simulink model "attitude3d"  (R2019b)
settings: Solver=ode4  StartTime=0.0  StopTime=6530  FixedStep=10  RelTol=1e-3
values from neighbouring files (symbols this model uses):
  antenna_vb = [1, 0, 0]    [attitude3d_init.m]
  init_xBI = [1, 0, 0]    [attitude3d_init.m]
  init_yBI = [0, 1, 0]    [attitude3d_init.m]
  init_zBI = [0, 0, 1]    [attitude3d_init.m]
  P = 2 * pi / mean_motion    [attitude3d_init.m]
  solar_array_vb = [1, 0, 0]    [attitude3d_init.m]
  star_sensor_1_vb = [1/sqrt(2), +1/sqrt(2), 0]    [attitude3d_init.m]
  star_sensor_2_vb = [1/sqrt(2), -1/sqrt(2), 0]    [attitude3d_init.m]
  target_mean_radius = mean_mars_radius    (= 3389500)    [attitude3d_init.m]
  thrust_no_shadow_weight = 1.0    (= 1)    [attitude3d_init.m]
  thrust_shadow_weight = 1.0    (= 1)    [attitude3d_init.m]
  thruster_vb = [-1, 0, 0]    [attitude3d_init.m]
  window_n = int16(window_t/10.0)    [attitude3d_init.m]
  x = [0,        max_omega*0.1,  0, 0               ;      0.5 * P,  max_omega*0.1,  0, 0               ;      1.0 * P,  max_omega*0.1,  0, 0               ]    [attitude3d_init.m]
libraries: vrlib x14, simulink x6, dspstat3 x4, commfilt2 x2
(part 1 of 2)
settings Model: Creator=ggarrett  LastModifiedBy=ggarrett
settings HardwareCC: TargetBitPerLong=64  TargetBitPerPointer=64  TargetBitPerSizeT=64  TargetBitPerPtrDiffT=64  TargetLongLongMode=on  TargetIntDivRoundTo=Zero  TargetEndianess=LittleEndian  TargetWordSize=64  TargetHWDeviceType=MATLAB Host  ProdEqTarget=off
settings RTWCC: Description=Rapid Simulation Target  SystemTargetFile=rsim.tlc  TemplateMakefile=rsim_default_tmf
settings RSimTargetCC: TargetLangStandard=C99 (ISO)  GeneratePreprocessorConditionals=Use local settings  PreserveStateflowLocalDataDimensions=off

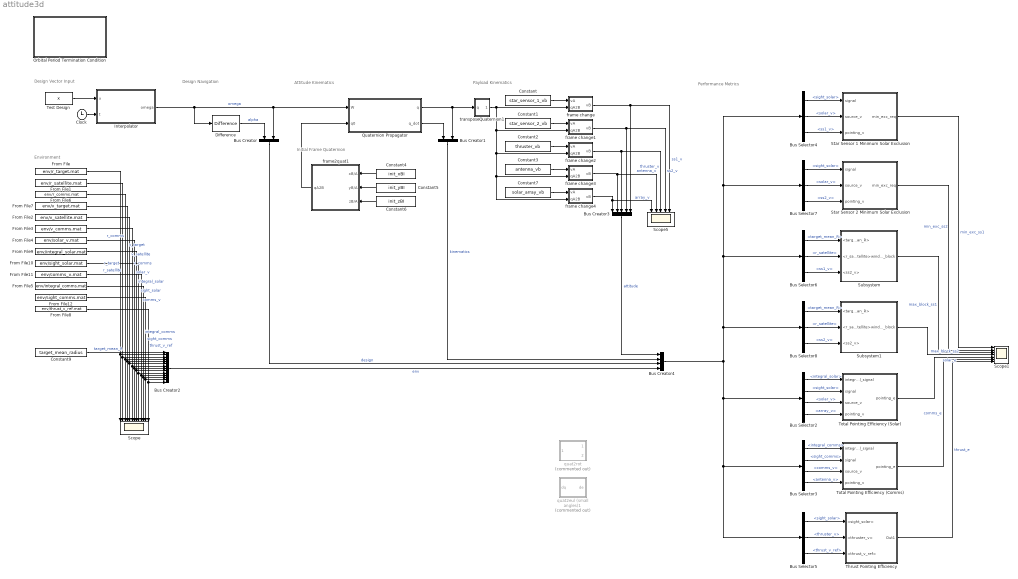
== system attitude3d ==
  note: Performance Metrics
  note: Attitude Kinematics
  note: Design Vector Input
  note: Design Navigation
  note: Payload Kinematics
  note: Environment
  note: Initial Frame Quaternion
  Bus Creator : BusCreator  Inputs=2
  Bus Creator1 : BusCreator  Inputs=2
  Bus Creator2 : BusCreator  Inputs=14
  Bus Creator3 : BusCreator  Inputs=5
  Bus Creator4 : BusCreator  Inputs=4
  Bus Selector2 : BusSelector  OutputSignals=env.integral_solar,env.sight_solar,env.solar_v,attitude.array_v
  Bus Selector3 : BusSelector  OutputSignals=env.integral_comms,env.sight_comms,env.comms_v,attitude.antenna_v
  Bus Selector4 : BusSelector  OutputSignals=env.sight_solar,env.solar_v,attitude.ss1_v
  Bus Selector5 : BusSelector  OutputSignals=env.sight_solar,attitude.thruster_v,env.thrust_v_ref
  Bus Selector6 : BusSelector  OutputSignals=env.target_mean_R,env.r_satellite,attitude.ss1_v
  Bus Selector7 : BusSelector  OutputSignals=env.sight_solar,env.solar_v,attitude.ss2_v
  Bus Selector8 : BusSelector  OutputSignals=env.target_mean_R,env.r_satellite,attitude.ss2_v
  Clock : Clock
  Constant : Constant  Value=star_sensor_1_vb
  Constant1 : Constant  Value=star_sensor_2_vb
  Constant2 : Constant  Value=thruster_vb
  Constant3 : Constant  Value=antenna_vb
  Constant4 : Constant  Value=init_xBI
  Constant5 : Constant  Value=init_yBI
  Constant6 : Constant  Value=init_zBI
  Constant7 : Constant  Value=solar_array_vb
  Constant9 : Constant  Value=target_mean_radius
  Difference : simulink/Discrete/Difference  ICPrevInput=0.0  OutMin=[]  OutMax=[]  OutDataType=fixdt(1, 16)  OutScaling=2^-10  DoSatur=off
  From File : FromFile  FileName=env/r_target.mat  SampleTime=0
  From File1 : FromFile  FileName=env/r_satellite.mat  SampleTime=0
  From File10 : FromFile  FileName=env/sight_solar.mat  SampleTime=0
  From File11 : FromFile  FileName=env/comms_v.mat  SampleTime=0
  From File12 : FromFile  FileName=env/sight_comms.mat  SampleTime=0
  From File2 : FromFile  FileName=env/v_satellite.mat  SampleTime=0
  From File3 : FromFile  FileName=env/v_comms.mat  SampleTime=0
  From File4 : FromFile  FileName=env/solar_v.mat  SampleTime=0
  From File5 : FromFile  FileName=env/integral_comms.mat  SampleTime=0
  From File6 : FromFile  FileName=env/r_comms.mat  SampleTime=0
  From File7 : FromFile  FileName=env/v_target.mat  SampleTime=0
  From File8 : FromFile  FileName=env/thrust_v_ref.mat  SampleTime=0
  From File9 : FromFile  FileName=env/integral_solar.mat  SampleTime=0
  "Interpolator " : MATLAB Function  TreatAsAtomicUnit=on
  Orbital Period Termination Condition : Subsystem
  Quaternion Propagator : Subsystem
  Scope : Scope  NumInputPorts=13
  Scope1 : Scope  NumInputPorts=7
  Scope5 : Scope  NumInputPorts=5
  Star Sensor 1 Minimum Solar Exclusion : Subsystem
  Star Sensor 2 Minimum Solar Exclusion : Subsystem
  Subsystem : Subsystem
  Subsystem1 : Subsystem
  Test Design : Constant  Value=x
  Thrust Pointing Efficiency : Subsystem
  Total Pointing Efficiency (Comms) : Subsystem
  Total Pointing Efficiency (Solar) : Subsystem
  frame change : Subsystem  mask(Frame change){inLabel=b, outLabel=i}
      mask prompts: inLabel "Label for initial frame"; outLabel "Label for target frame"
      mask help: Express input vector in frame B, using the quaternion describing the rotation from frame A to frame B.
      mask Display:
      | port_label('input',1,['v',inLabel]);
      | port_label('output',1,['v',outLabel]);
      | port_label('input',2,['q',inLabel,'2',outLabel]);
  frame change1 : Subsystem  mask(Frame change){inLabel=b, outLabel=i}
      mask prompts: inLabel "Label for initial frame"; outLabel "Label for target frame"
      mask help: Express input vector in frame B, using the quaternion describing the rotation from frame A to frame B.
      mask Display:
      | port_label('input',1,['v',inLabel]);
      | port_label('output',1,['v',outLabel]);
      | port_label('input',2,['q',inLabel,'2',outLabel]);
  frame change2 : Subsystem  mask(Frame change){inLabel=b, outLabel=i}
      mask prompts: inLabel "Label for initial frame"; outLabel "Label for target frame"
      mask help: Express input vector in frame B, using the quaternion describing the rotation from frame A to frame B.
      mask Display:
      | port_label('input',1,['v',inLabel]);
      | port_label('output',1,['v',outLabel]);
      | port_label('input',2,['q',inLabel,'2',outLabel]);
  frame change3 : Subsystem  mask(Frame change){inLabel=b, outLabel=i}
      mask prompts: inLabel "Label for initial frame"; outLabel "Label for target frame"
      mask help: Express input vector in frame B, using the quaternion describing the rotation from frame A to frame B.
      mask Display:
      | port_label('input',1,['v',inLabel]);
      | port_label('output',1,['v',outLabel]);
      | port_label('input',2,['q',inLabel,'2',outLabel]);
  frame change4 : Subsystem  mask(Frame change){inLabel=b, outLabel=i}
      mask prompts: inLabel "Label for initial frame"; outLabel "Label for target frame"
      mask help: Express input vector in frame B, using the quaternion describing the rotation from frame A to frame B.
      mask Display:
      | port_label('input',1,['v',inLabel]);
      | port_label('output',1,['v',outLabel]);
      | port_label('input',2,['q',inLabel,'2',outLabel]);
  frame2quat1 : Subsystem  mask(Compute quaternion from 3 orthogonal unit vectors){Alabel=I, Blabel=B}
      mask prompts: Alabel "Label for origin frame"; Blabel "Label for target frame"
      mask help: Determines the attitude quaternion representing the rotation which transforms the origin frame into the target frame, from the unit vectors of target frame expressed in origin frame.
      mask Display:
      | port_label('input',1,['x',Blabel,'/',Alabel]);
      | port_label('input',2,['y',Blabel,'/',Alabel]);
      | port_label('input',3,['z',Blabel,'/',Alabel]);
      | port_label('output',1,['q',Alabel,'2',Blabel]);
  quat2eul (small angles)1 : Subsystem  Commented=on  mask(Small quat error to small angles error){}
      mask help:
      | [dphi,dtheta,dpsi] = u*dTheta
      | where
      | dq = [cos(dTheta/2); u*sin(dTheta/2)]
  quat2rot : Subsystem  Commented=on  mask(Find axis and angle from quaternion){Alabel=I, Blabel=B}
      mask prompts: Alabel "Label for origin frame"; Blabel "Label for target frame"
      mask help: Extracts the axis (unit vector) and angle (rad) of the rotation from origin frame to target frame, from the quaternion representing that rotation
      mask Display:
      | port_label('input',1,['q',Alabel,'2',Blabel]);
      | port_label('output',1,['th_',Alabel,'2',Blabel]);
      | port_label('output',2,['u_',Alabel]);
  transposeQuaternion1 : Subsystem  mask(transposeQuaternion){}
      mask help:
      | Compute the transpose (inverse or conjugate) of the input quaternion
      |
      | Inputs:
      |   q     Quaternion
      |
      | Outputs:
      |   qt     Transpose of the input quaternion
      mask Help: eval('starDoc simulink/transposeQuaternion');
      mask Display: disp('q''');
  wires:
  Test Design/1 -> "Interpolator "/1(x)
  Clock/1 -> "Interpolator "/2(t)
  From File/1 -> Scope/1, Bus Creator2/2  "r_target"
  From File1/1 -> Scope/2, Bus Creator2/3  "r_satellite"
  From File6/1 -> Scope/3, Bus Creator2/4  "r_comms"
  From File7/1 -> Scope/4, Bus Creator2/5  "v_target"
  From File2/1 -> Scope/5, Bus Creator2/6  "v_satellite"
  From File3/1 -> Scope/6, Bus Creator2/7  "v_comms"
  From File4/1 -> Scope/7, Bus Creator2/8  "solar_v"
  "Interpolator "/1(omega) -> Difference/1, Quaternion Propagator/1(W), Bus Creator/2  "omega"
  Difference/1 -> Bus Creator/1  "alpha"
  Quaternion Propagator/2(q_dot) -> Bus Creator1/1
  Constant/1 -> frame change/1(vA)
  Constant1/1 -> frame change1/1(vA)
  Constant2/1 -> frame change2/1(vA)
  Constant3/1 -> frame change3/1(vA)
  Bus Creator/1 -> Bus Creator4/3  "design"
  Bus Creator1/1 -> Bus Creator4/2  "kinematics"
  Bus Creator2/1 -> Bus Creator4/4  "env"
  Constant5/1 -> frame2quat1/2(yB/A)
  Quaternion Propagator/1(q) -> transposeQuaternion1/1(q), Bus Creator1/2
  Constant6/1 -> frame2quat1/3(zB/A)
  Constant4/1 -> frame2quat1/1(xB/A)
  frame2quat1/1(qA2B) -> Quaternion Propagator/2(q0)
  frame change/1(vB) -> Scope5/5, Bus Creator3/5  "ss1_v"
  frame change1/1(vB) -> Scope5/4, Bus Creator3/4  "ss2_v"
  frame change2/1(vB) -> Scope5/3, Bus Creator3/3  "thruster_v"
  frame change3/1(vB) -> Scope5/2, Bus Creator3/2  "antenna_v"
  Bus Creator3/1 -> Bus Creator4/1  "attitude"
  Constant7/1 -> frame change4/1(vA)
  transposeQuaternion1/1(q') -> frame change4/2(qA2B), frame change3/2(qA2B), frame change2/2(qA2B), frame change1/2(qA2B), frame change/2(qA2B)
  frame change4/1(vB) -> Scope5/1, Bus Creator3/1  "array_v"
  Bus Creator4/1 -> Bus Selector4/1, Bus Selector7/1, Bus Selector6/1, Bus Selector8/1, Bus Selector5/1, Bus Selector3/1, Bus Selector2/1
  From File9/1 -> Scope/8, Bus Creator2/9  "integral_solar"
  From File10/1 -> Scope/9, Bus Creator2/10  "sight_solar"
  From File11/1 -> Scope/10, Bus Creator2/11  "comms_v"
  From File5/1 -> Scope/11, Bus Creator2/12  "integral_comms"
  From File12/1 -> Scope/12, Bus Creator2/13  "sight_comms"
  Bus Selector2/3 -> Total Pointing Efficiency (Solar)/3(source_v)  "<solar_v>"
  Bus Selector2/4 -> Total Pointing Efficiency (Solar)/4(pointing_v)  "<array_v>"
  Bus Selector2/1 -> Total Pointing Efficiency (Solar)/1(integral_signal)  "<integral_solar>"
  Bus Selector2/2 -> Total Pointing Efficiency (Solar)/2(signal)  "<sight_solar>"
  Bus Selector3/4 -> Total Pointing Efficiency (Comms)/4(pointing_v)  "<antenna_v>"
  Bus Selector3/1 -> Total Pointing Efficiency (Comms)/1(integral_signal)  "<integral_comms>"
  Bus Selector3/3 -> Total Pointing Efficiency (Comms)/3(source_v)  "<comms_v>"
  Bus Selector3/2 -> Total Pointing Efficiency (Comms)/2(signal)  "<sight_comms>"
  Bus Selector4/3 -> Star Sensor 1 Minimum Solar Exclusion/3(pointing_v)  "<ss1_v>"
  Bus Selector4/1 -> Star Sensor 1 Minimum Solar Exclusion/1(signal)  "<sight_solar>"
  Bus Selector4/2 -> Star Sensor 1 Minimum Solar Exclusion/2(source_v)  "<solar_v>"
  From File8/1 -> Bus Creator2/14, Scope/13  "thrust_v_ref"
  Bus Selector5/1 -> Thrust Pointing Efficiency/1(<sight_solar>)  "<sight_solar>"
  Bus Selector5/2 -> Thrust Pointing Efficiency/2(<thruster_v>)  "<thruster_v>"
  Bus Selector5/3 -> Thrust Pointing Efficiency/3(<thrust_v_ref>)  "<thrust_v_ref>"
  Bus Selector7/3 -> Star Sensor 2 Minimum Solar Exclusion/3(pointing_v)  "<ss2_v>"
  Bus Selector7/1 -> Star Sensor 2 Minimum Solar Exclusion/1(signal)  "<sight_solar>"
  Bus Selector7/2 -> Star Sensor 2 Minimum Solar Exclusion/2(source_v)  "<solar_v>"
  Constant9/1 -> Bus Creator2/1  "target_mean_R"
  Bus Selector6/1 -> Subsystem/1(<target_mean_R>)  "<target_mean_R>"
  Bus Selector6/2 -> Subsystem/2(<r_satellite>)  "<r_satellite>"
  Bus Selector6/3 -> Subsystem/3(<ss2_v>)  "<ss1_v>"
  Bus Selector8/1 -> Subsystem1/1(<target_mean_R>)  "<target_mean_R>"
  Bus Selector8/2 -> Subsystem1/2(<r_satellite>)  "<r_satellite>"
  Bus Selector8/3 -> Subsystem1/3(<ss2_v>)  "<ss2_v>"
  Subsystem1/1(window_block) -> Scope1/4  "max_block_ss2"
  Subsystem/1(window_block) -> Scope1/3  "max_block_ss1"
  Star Sensor 2 Minimum Solar Exclusion/1(min_exc_req) -> Scope1/2  "min_exc_ss2"
  Star Sensor 1 Minimum Solar Exclusion/1(min_exc_req) -> Scope1/1  "min_exc_ss1"
  Total Pointing Efficiency (Solar)/1(pointing_e) -> Scope1/5  "solar_e"
  Total Pointing Efficiency (Comms)/1(pointing_e) -> Scope1/6  "comms_e"
  Thrust Pointing Efficiency/1(Out1) -> Scope1/7  "thrust_e"

== system attitude3d/Orbital Period Termination Condition ==
  Clock1 : Clock
  Compare To Zero : simulink/Logic and Bit Operations/Compare To Zero  relop=<=  OutDataTypeStr=boolean
  Constant : Constant  Value=0.997*P
  Scope : Scope  NumInputPorts=2
  Stop Simulation : Stop
  Sum : Sum  Inputs=|-+
  wires:
  Constant/1 -> Scope/1, Sum/2
  Clock1/1 -> Scope/2, Sum/1
  Sum/1 -> Compare To Zero/1
  Compare To Zero/1 -> Stop Simulation/1

== system attitude3d/Quaternion Propagator ==
  W : Inport
  q0 : Inport  Port=2
  Integrator : Integrator  InitialConditionSource=external
  Quaternion Differential : MATLAB Function  TreatAsAtomicUnit=on
  Quaternion Normed : MATLAB Function  TreatAsAtomicUnit=on
  Scope : Scope  NumInputPorts=2
  q : Outport
  q_dot : Outport  Port=2
  wires:
  Integrator/1 -> Quaternion Normed/1(u)
  q0/1 -> Integrator/2
  Quaternion Differential/1(q_dot) -> q_dot/1, Integrator/1, Scope/2
  W/1 -> Quaternion Differential/2(omega)
  Quaternion Normed/1(y) -> Quaternion Differential/1(q), Scope/1, q/1

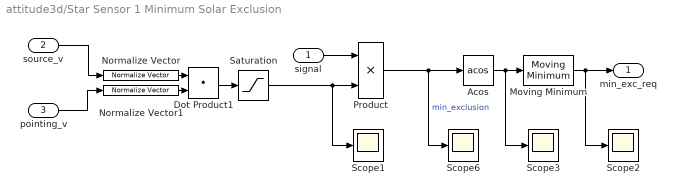
== system attitude3d/Star Sensor 1 Minimum Solar Exclusion ==
  signal : Inport
  source_v : Inport  Port=2
  pointing_v : Inport  Port=3
  Acos : Trigonometry  Operator=acos
  Dot Product1 : DotProduct  InputSameDT=on  OutDataTypeStr=Inherit: Inherit via internal rule
  Moving Minimum : dspstat3/Moving Minimum  SpecifyWindowLength=off  WindowLength=int16(P/10)  SimulateUsing=Code generation
      settings: SourceProductName=DSP System Toolbox  SourceProductBaseCode=DS
  Normalize Vector : vrlib/Utilities/Normalize Vector  maxzero=0
      settings: SourceProductName=Simulink
  Normalize Vector1 : vrlib/Utilities/Normalize Vector  maxzero=0
      settings: SourceProductName=Simulink
  Product : Product
  Saturation : Saturate  UpperLimit=1.0  LowerLimit=0
  Scope{1..3,6} (4 alike) : Scope
  min_exc_req : Outport
  wires:
  Dot Product1/1 -> Saturation/1
  Normalize Vector1/1 -> Dot Product1/2
  signal/1 -> Product/1
  source_v/1 -> Normalize Vector/1
  pointing_v/1 -> Normalize Vector1/1
  Normalize Vector/1 -> Dot Product1/1
  Saturation/1 -> Scope1/1, Product/2
  Product/1 -> Scope6/1, Acos/1  "min_exclusion"
  Acos/1 -> Scope3/1, Moving Minimum/1
  Moving Minimum/1 -> Scope2/1, min_exc_req/1

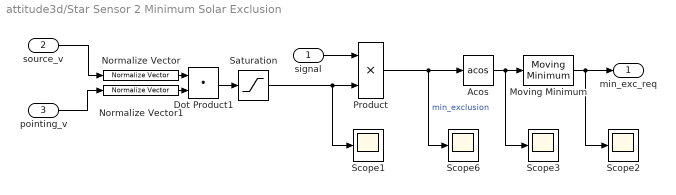
== system attitude3d/Star Sensor 2 Minimum Solar Exclusion ==
  signal : Inport
  source_v : Inport  Port=2
  pointing_v : Inport  Port=3
  Acos : Trigonometry  Operator=acos
  Dot Product1 : DotProduct  InputSameDT=on  OutDataTypeStr=Inherit: Inherit via internal rule
  Moving Minimum : dspstat3/Moving Minimum  SpecifyWindowLength=off  WindowLength=int16(P/10)  SimulateUsing=Code generation
      settings: SourceProductName=DSP System Toolbox  SourceProductBaseCode=DS
  Normalize Vector : vrlib/Utilities/Normalize Vector  maxzero=0
      settings: SourceProductName=Simulink
  Normalize Vector1 : vrlib/Utilities/Normalize Vector  maxzero=0
      settings: SourceProductName=Simulink
  Product : Product
  Saturation : Saturate  UpperLimit=1.0  LowerLimit=0
  Scope{1..3,6} (4 alike) : Scope
  min_exc_req : Outport
  wires:
  Dot Product1/1 -> Saturation/1
  Normalize Vector1/1 -> Dot Product1/2
  signal/1 -> Product/1
  source_v/1 -> Normalize Vector/1
  pointing_v/1 -> Normalize Vector1/1
  Normalize Vector/1 -> Dot Product1/1
  Saturation/1 -> Scope1/1, Product/2
  Product/1 -> Scope6/1, Acos/1  "min_exclusion"
  Acos/1 -> Scope3/1, Moving Minimum/1
  Moving Minimum/1 -> Scope2/1, min_exc_req/1

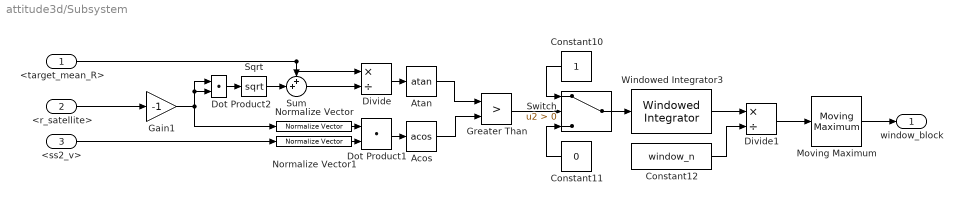
== system attitude3d/Subsystem ==
  <target_mean_R> : Inport
  <r_satellite> : Inport  Port=2
  <ss2_v> : Inport  Port=3
  Acos : Trigonometry  Operator=acos
  Atan : Trigonometry  Operator=atan
  Constant10 : Constant
  Constant11 : Constant  Value=0
  Constant12 : Constant  Value=window_n
  Divide : Product  Inputs=*/
  Divide1 : Product  Inputs=*/
  Dot Product1 : DotProduct  InputSameDT=on  OutDataTypeStr=Inherit: Inherit via internal rule
  Dot Product2 : DotProduct  InputSameDT=on  OutDataTypeStr=Inherit: Inherit via internal rule
  Gain1 : Gain  Gain=-1
  Greater Than : RelationalOperator  Operator=>  OutDataTypeStr=boolean  RndMeth=Simplest
  Moving Maximum : dspstat3/Moving Maximum  SpecifyWindowLength=on  WindowLength=4  SimulateUsing=Code generation
      settings: SourceProductName=DSP System Toolbox  SourceProductBaseCode=DS
  Normalize Vector : vrlib/Utilities/Normalize Vector  maxzero=0
      settings: SourceProductName=Simulink
  Normalize Vector1 : vrlib/Utilities/Normalize Vector  maxzero=0
      settings: SourceProductName=Simulink
  Sqrt : Sqrt  SaturateOnIntegerOverflow=on
  Sum : Sum  Inputs=++|
  Switch : Switch  Criteria=u2 > Threshold
  Windowed Integrator3 : commfilt2/Windowed Integrator  integperiod=window_n  InputProcessing=Columns as channels (frame based)  roundingMode=Floor  overflowMode=off  coeffDataTypeStr=Inherit: Same word length as input  coeffMin=[]  coeffMax=[]  coeffLastDataTypeStr=Inherit: Same word length as input  accumDataTypeStr=Inherit: Same as product output  accumLastDataTypeStr=Inherit: Same as product output  outputDataTypeStr=Inherit: Same as accumulator  outputMin=[]  outputMax=[]  outputLastDataTypeStr=Inherit: Same as accumulator
      settings: SourceProductName=Communications Toolbox  SourceProductBaseCode=CM
  window_block : Outport
  wires:
  Sum/1 -> Divide/2
  Dot Product1/1 -> Acos/1
  Normalize Vector/1 -> Dot Product1/1
  Divide1/1 -> Moving Maximum/1
  Constant12/1 -> Divide1/2
  Divide/1 -> Atan/1
  Atan/1 -> Greater Than/1
  Dot Product2/1 -> Sqrt/1
  Moving Maximum/1 -> window_block/1
  Acos/1 -> Greater Than/2
  <r_satellite>/1 -> Gain1/1
  <ss2_v>/1 -> Normalize Vector1/1
  Normalize Vector1/1 -> Dot Product1/2
  Sqrt/1 -> Sum/2
  Constant11/1 -> Switch/3
  Constant10/1 -> Switch/1
  Greater Than/1 -> Switch/2
  <target_mean_R>/1 -> Divide/1, Sum/1
  Gain1/1 -> Normalize Vector/1, Dot Product2/1, Dot Product2/2
  Windowed Integrator3/1 -> Divide1/1
  Switch/1 -> Windowed Integrator3/1

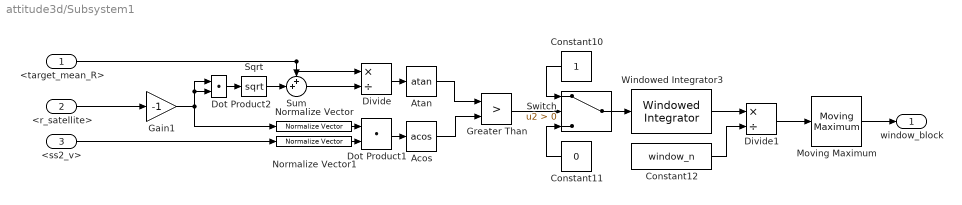
== system attitude3d/Subsystem1 ==
  <target_mean_R> : Inport
  <r_satellite> : Inport  Port=2
  <ss2_v> : Inport  Port=3
  Acos : Trigonometry  Operator=acos
  Atan : Trigonometry  Operator=atan
  Constant10 : Constant
  Constant11 : Constant  Value=0
  Constant12 : Constant  Value=window_n
  Divide : Product  Inputs=*/
  Divide1 : Product  Inputs=*/
  Dot Product1 : DotProduct  InputSameDT=on  OutDataTypeStr=Inherit: Inherit via internal rule
  Dot Product2 : DotProduct  InputSameDT=on  OutDataTypeStr=Inherit: Inherit via internal rule
  Gain1 : Gain  Gain=-1
  Greater Than : RelationalOperator  Operator=>  OutDataTypeStr=boolean  RndMeth=Simplest
  Moving Maximum : dspstat3/Moving Maximum  SpecifyWindowLength=on  WindowLength=4  SimulateUsing=Code generation
      settings: SourceProductName=DSP System Toolbox  SourceProductBaseCode=DS
  Normalize Vector : vrlib/Utilities/Normalize Vector  maxzero=0
      settings: SourceProductName=Simulink
  Normalize Vector1 : vrlib/Utilities/Normalize Vector  maxzero=0
      settings: SourceProductName=Simulink
  Sqrt : Sqrt  SaturateOnIntegerOverflow=on
  Sum : Sum  Inputs=++|
  Switch : Switch  Criteria=u2 > Threshold
  Windowed Integrator3 : commfilt2/Windowed Integrator  integperiod=window_n  InputProcessing=Columns as channels (frame based)  roundingMode=Floor  overflowMode=off  coeffDataTypeStr=Inherit: Same word length as input  coeffMin=[]  coeffMax=[]  coeffLastDataTypeStr=Inherit: Same word length as input  accumDataTypeStr=Inherit: Same as product output  accumLastDataTypeStr=Inherit: Same as product output  outputDataTypeStr=Inherit: Same as accumulator  outputMin=[]  outputMax=[]  outputLastDataTypeStr=Inherit: Same as accumulator
      settings: SourceProductName=Communications Toolbox  SourceProductBaseCode=CM
  window_block : Outport
  wires:
  Sum/1 -> Divide/2
  Dot Product1/1 -> Acos/1
  Normalize Vector/1 -> Dot Product1/1
  Divide1/1 -> Moving Maximum/1
  Constant12/1 -> Divide1/2
  Divide/1 -> Atan/1
  Atan/1 -> Greater Than/1
  Dot Product2/1 -> Sqrt/1
  Moving Maximum/1 -> window_block/1
  Acos/1 -> Greater Than/2
  <r_satellite>/1 -> Gain1/1
  <ss2_v>/1 -> Normalize Vector1/1
  Normalize Vector1/1 -> Dot Product1/2
  Sqrt/1 -> Sum/2
  Constant11/1 -> Switch/3
  Constant10/1 -> Switch/1
  Greater Than/1 -> Switch/2
  <target_mean_R>/1 -> Divide/1, Sum/1
  Gain1/1 -> Normalize Vector/1, Dot Product2/1, Dot Product2/2
  Windowed Integrator3/1 -> Divide1/1
  Switch/1 -> Windowed Integrator3/1

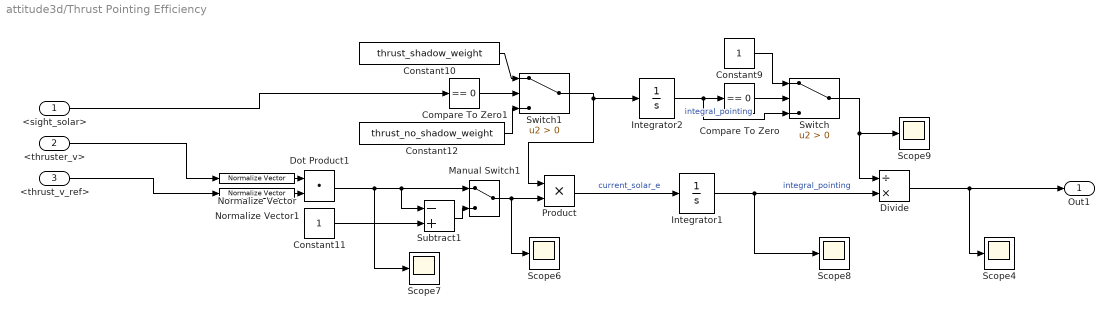
== system attitude3d/Thrust Pointing Efficiency ==
  <sight_solar> : Inport
  <thruster_v> : Inport  Port=2
  <thrust_v_ref> : Inport  Port=3
  Compare To Zero : simulink/Logic and Bit Operations/Compare To Zero  relop===  OutDataTypeStr=boolean
  Compare To Zero1 : simulink/Logic and Bit Operations/Compare To Zero  relop===  OutDataTypeStr=boolean
  Constant10 : Constant  Value=thrust_shadow_weight
  Constant11 : Constant
  Constant12 : Constant  Value=thrust_no_shadow_weight
  Constant9 : Constant
  Divide : Product  Inputs=/*
  Dot Product1 : DotProduct  InputSameDT=on  OutDataTypeStr=Inherit: Inherit via internal rule
  Integrator1 : Integrator
  Integrator2 : Integrator
  Manual Switch1 : ManualSwitch
  Normalize Vector : vrlib/Utilities/Normalize Vector  maxzero=0
      settings: SourceProductName=Simulink
  Normalize Vector1 : vrlib/Utilities/Normalize Vector  maxzero=0
      settings: SourceProductName=Simulink
  Product : Product
  Scope{4,6..9} (5 alike) : Scope
  Subtract1 : Sum  Inputs=-+
  Switch : Switch  Criteria=u2 > Threshold
  Switch1 : Switch  Criteria=u2 > Threshold
  Out1 : Outport
  wires:
  Constant9/1 -> Switch/1
  Normalize Vector/1 -> Dot Product1/1
  Product/1 -> Integrator1/1  "current_solar_e"
  Compare To Zero1/1 -> Switch1/2
  Constant12/1 -> Switch1/3
  Manual Switch1/1 -> Scope6/1, Product/2
  Dot Product1/1 -> Scope7/1, Subtract1/1, Manual Switch1/1
  Integrator1/1 -> Scope8/1, Divide/2  "integral_pointing"
  Switch/1 -> Scope9/1, Divide/1
  Integrator2/1 -> Switch/3, Compare To Zero/1  "integral_pointing"
  Normalize Vector1/1 -> Dot Product1/2
  Constant10/1 -> Switch1/1
  Constant11/1 -> Subtract1/2
  Divide/1 -> Out1/1, Scope4/1
  <sight_solar>/1 -> Compare To Zero1/1
  Subtract1/1 -> Manual Switch1/2
  <thrust_v_ref>/1 -> Normalize Vector1/1
  Compare To Zero/1 -> Switch/2
  Switch1/1 -> Integrator2/1, Product/1
  <thruster_v>/1 -> Normalize Vector/1

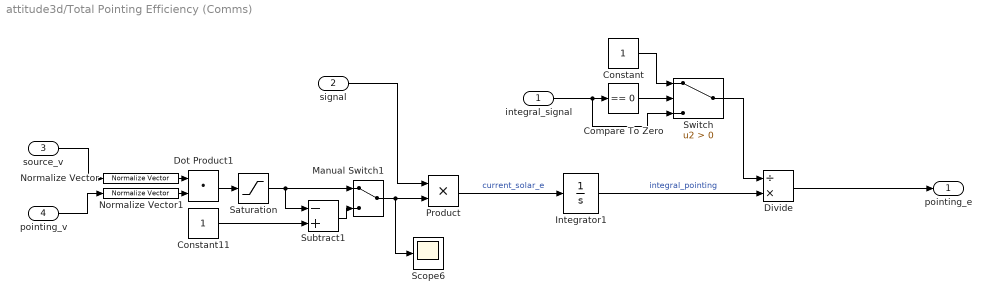
== system attitude3d/Total Pointing Efficiency (Comms) ==
  integral_signal : Inport
  signal : Inport  Port=2
  source_v : Inport  Port=3
  pointing_v : Inport  Port=4
  Compare To Zero : simulink/Logic and Bit Operations/Compare To Zero  relop===  OutDataTypeStr=boolean
  Constant : Constant
  Constant11 : Constant
  Divide : Product  Inputs=/*
  Dot Product1 : DotProduct  InputSameDT=on  OutDataTypeStr=Inherit: Inherit via internal rule
  Integrator1 : Integrator
  Manual Switch1 : ManualSwitch
  Normalize Vector : vrlib/Utilities/Normalize Vector  maxzero=0
      settings: SourceProductName=Simulink
  Normalize Vector1 : vrlib/Utilities/Normalize Vector  maxzero=0
      settings: SourceProductName=Simulink
  Product : Product
  Saturation : Saturate  UpperLimit=1.0  LowerLimit=0
  Scope6 : Scope
  Subtract1 : Sum  Inputs=-+
  Switch : Switch  Criteria=u2 > Threshold
  pointing_e : Outport
  wires:
  Subtract1/1 -> Manual Switch1/2
  Dot Product1/1 -> Saturation/1
  Normalize Vector1/1 -> Dot Product1/2
  Saturation/1 -> Subtract1/1, Manual Switch1/1
  Product/1 -> Integrator1/1  "current_solar_e"
  integral_signal/1 -> Switch/3, Compare To Zero/1
  signal/1 -> Product/1
  source_v/1 -> Normalize Vector/1
  Constant11/1 -> Subtract1/2
  Manual Switch1/1 -> Scope6/1, Product/2
  Divide/1 -> pointing_e/1
  pointing_v/1 -> Normalize Vector1/1
  Integrator1/1 -> Divide/2  "integral_pointing"
  Normalize Vector/1 -> Dot Product1/1
  Compare To Zero/1 -> Switch/2
  Constant/1 -> Switch/1
  Switch/1 -> Divide/1

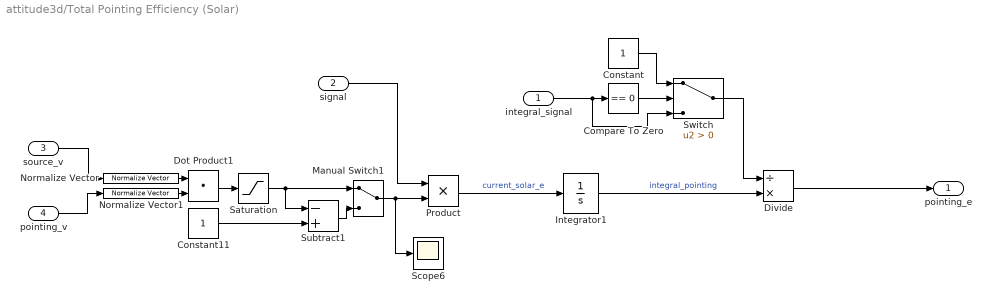
== system attitude3d/Total Pointing Efficiency (Solar) ==
  integral_signal : Inport
  signal : Inport  Port=2
  source_v : Inport  Port=3
  pointing_v : Inport  Port=4
  Compare To Zero : simulink/Logic and Bit Operations/Compare To Zero  relop===  OutDataTypeStr=boolean
  Constant : Constant
  Constant11 : Constant
  Divide : Product  Inputs=/*
  Dot Product1 : DotProduct  InputSameDT=on  OutDataTypeStr=Inherit: Inherit via internal rule
  Integrator1 : Integrator
  Manual Switch1 : ManualSwitch
  Normalize Vector : vrlib/Utilities/Normalize Vector  maxzero=0
      settings: SourceProductName=Simulink
  Normalize Vector1 : vrlib/Utilities/Normalize Vector  maxzero=0
      settings: SourceProductName=Simulink
  Product : Product
  Saturation : Saturate  UpperLimit=1.0  LowerLimit=0
  Scope6 : Scope
  Subtract1 : Sum  Inputs=-+
  Switch : Switch  Criteria=u2 > Threshold
  pointing_e : Outport
  wires:
  Subtract1/1 -> Manual Switch1/2
  Dot Product1/1 -> Saturation/1
  Normalize Vector1/1 -> Dot Product1/2
  Saturation/1 -> Subtract1/1, Manual Switch1/1
  Product/1 -> Integrator1/1  "current_solar_e"
  integral_signal/1 -> Switch/3, Compare To Zero/1
  signal/1 -> Product/1
  source_v/1 -> Normalize Vector/1
  Constant11/1 -> Subtract1/2
  Manual Switch1/1 -> Scope6/1, Product/2
  Divide/1 -> pointing_e/1
  pointing_v/1 -> Normalize Vector1/1
  Integrator1/1 -> Divide/2  "integral_pointing"
  Normalize Vector/1 -> Dot Product1/1
  Compare To Zero/1 -> Switch/2
  Constant/1 -> Switch/1
  Switch/1 -> Divide/1

== system attitude3d/frame change ==
  vA : Inport
  qA2B : Inport  Port=2
  Constant : Constant
  Demux : Demux  Outputs=[1 3]
  Mux : Mux  Inputs=2
  Product : Product  Inputs=/*  SaturateOnIntegerOverflow=on  OutDataTypeStr=Inherit: Same as first input
  quat product : Subsystem
      mask Display:
      | plot(0.5+cos(linspace(0,2*pi,65))*0.3,0.5+sin(linspace(0,2*pi,65))*0.3);
      | plot([.29 .71],[.29 .71]);
      | plot([.71 .29],[.29 .71]);
  quat product1 : Subsystem
      mask Display:
      | plot(0.5+cos(linspace(0,2*pi,65))*0.3,0.5+sin(linspace(0,2*pi,65))*0.3);
      | plot([.29 .71],[.29 .71]);
      | plot([.71 .29],[.29 .71]);
  transposeQuaternion : Subsystem  mask(transposeQuaternion){}
      mask help:
      | Compute the transpose (inverse or conjugate) of the input quaternion
      |
      | Inputs:
      |   q     Quaternion
      |
      | Outputs:
      |   qt     Transpose of the input quaternion
      mask Help: eval('starDoc simulink/transposeQuaternion');
      mask Display: disp('q''');
  vB : Outport
  wires:
  Product/1 -> vB/1
  quat product1/1(q1*q2) -> Demux/1
  quat product/1(q1*q2) -> quat product1/1(q1)
  Mux/1 -> quat product/2(q2)
  transposeQuaternion/1(q') -> quat product/1(q1)
  qA2B/1 -> quat product1/2(q2), transposeQuaternion/1(q)
  vA/1 -> Mux/2
  Constant/1 -> Mux/1
  Demux/1 -> Product/1
  Demux/2 -> Product/2

== system attitude3d/frame change1 ==
  vA : Inport
  qA2B : Inport  Port=2
  Constant : Constant
  Demux : Demux  Outputs=[1 3]
  Mux : Mux  Inputs=2
  Product : Product  Inputs=/*  SaturateOnIntegerOverflow=on  OutDataTypeStr=Inherit: Same as first input
  quat product : Subsystem
      mask Display:
      | plot(0.5+cos(linspace(0,2*pi,65))*0.3,0.5+sin(linspace(0,2*pi,65))*0.3);
      | plot([.29 .71],[.29 .71]);
      | plot([.71 .29],[.29 .71]);
  quat product1 : Subsystem
      mask Display:
      | plot(0.5+cos(linspace(0,2*pi,65))*0.3,0.5+sin(linspace(0,2*pi,65))*0.3);
      | plot([.29 .71],[.29 .71]);
      | plot([.71 .29],[.29 .71]);
  transposeQuaternion : Subsystem  mask(transposeQuaternion){}
      mask help:
      | Compute the transpose (inverse or conjugate) of the input quaternion
      |
      | Inputs:
      |   q     Quaternion
      |
      | Outputs:
      |   qt     Transpose of the input quaternion
      mask Help: eval('starDoc simulink/transposeQuaternion');
      mask Display: disp('q''');
  vB : Outport
  wires:
  Product/1 -> vB/1
  quat product1/1(q1*q2) -> Demux/1
  quat product/1(q1*q2) -> quat product1/1(q1)
  Mux/1 -> quat product/2(q2)
  transposeQuaternion/1(q') -> quat product/1(q1)
  qA2B/1 -> quat product1/2(q2), transposeQuaternion/1(q)
  vA/1 -> Mux/2
  Constant/1 -> Mux/1
  Demux/1 -> Product/1
  Demux/2 -> Product/2

== system attitude3d/frame change2 ==
  vA : Inport
  qA2B : Inport  Port=2
  Constant : Constant
  Demux : Demux  Outputs=[1 3]
  Mux : Mux  Inputs=2
  Product : Product  Inputs=/*  SaturateOnIntegerOverflow=on  OutDataTypeStr=Inherit: Same as first input
  quat product : Subsystem
      mask Display:
      | plot(0.5+cos(linspace(0,2*pi,65))*0.3,0.5+sin(linspace(0,2*pi,65))*0.3);
      | plot([.29 .71],[.29 .71]);
      | plot([.71 .29],[.29 .71]);
  quat product1 : Subsystem
      mask Display:
      | plot(0.5+cos(linspace(0,2*pi,65))*0.3,0.5+sin(linspace(0,2*pi,65))*0.3);
      | plot([.29 .71],[.29 .71]);
      | plot([.71 .29],[.29 .71]);
  transposeQuaternion : Subsystem  mask(transposeQuaternion){}
      mask help:
      | Compute the transpose (inverse or conjugate) of the input quaternion
      |
      | Inputs:
      |   q     Quaternion
      |
      | Outputs:
      |   qt     Transpose of the input quaternion
      mask Help: eval('starDoc simulink/transposeQuaternion');
      mask Display: disp('q''');
  vB : Outport
  wires:
  Product/1 -> vB/1
  quat product1/1(q1*q2) -> Demux/1
  quat product/1(q1*q2) -> quat product1/1(q1)
  Mux/1 -> quat product/2(q2)
  transposeQuaternion/1(q') -> quat product/1(q1)
  qA2B/1 -> quat product1/2(q2), transposeQuaternion/1(q)
  vA/1 -> Mux/2
  Constant/1 -> Mux/1
  Demux/1 -> Product/1
  Demux/2 -> Product/2

== system attitude3d/frame change3 ==
  vA : Inport
  qA2B : Inport  Port=2
  Constant : Constant
  Demux : Demux  Outputs=[1 3]
  Mux : Mux  Inputs=2
  Product : Product  Inputs=/*  SaturateOnIntegerOverflow=on  OutDataTypeStr=Inherit: Same as first input
  quat product : Subsystem
      mask Display:
      | plot(0.5+cos(linspace(0,2*pi,65))*0.3,0.5+sin(linspace(0,2*pi,65))*0.3);
      | plot([.29 .71],[.29 .71]);
      | plot([.71 .29],[.29 .71]);
  quat product1 : Subsystem
      mask Display:
      | plot(0.5+cos(linspace(0,2*pi,65))*0.3,0.5+sin(linspace(0,2*pi,65))*0.3);
      | plot([.29 .71],[.29 .71]);
      | plot([.71 .29],[.29 .71]);
  transposeQuaternion : Subsystem  mask(transposeQuaternion){}
      mask help:
      | Compute the transpose (inverse or conjugate) of the input quaternion
      |
      | Inputs:
      |   q     Quaternion
      |
      | Outputs:
      |   qt     Transpose of the input quaternion
      mask Help: eval('starDoc simulink/transposeQuaternion');
      mask Display: disp('q''');
  vB : Outport
  wires:
  Product/1 -> vB/1
  quat product1/1(q1*q2) -> Demux/1
  quat product/1(q1*q2) -> quat product1/1(q1)
  Mux/1 -> quat product/2(q2)
  transposeQuaternion/1(q') -> quat product/1(q1)
  qA2B/1 -> quat product1/2(q2), transposeQuaternion/1(q)
  vA/1 -> Mux/2
  Constant/1 -> Mux/1
  Demux/1 -> Product/1
  Demux/2 -> Product/2

== system attitude3d/frame change4 ==
  vA : Inport
  qA2B : Inport  Port=2
  Constant : Constant
  Demux : Demux  Outputs=[1 3]
  Mux : Mux  Inputs=2
  Product : Product  Inputs=/*  SaturateOnIntegerOverflow=on  OutDataTypeStr=Inherit: Same as first input
  quat product : Subsystem
      mask Display:
      | plot(0.5+cos(linspace(0,2*pi,65))*0.3,0.5+sin(linspace(0,2*pi,65))*0.3);
      | plot([.29 .71],[.29 .71]);
      | plot([.71 .29],[.29 .71]);
  quat product1 : Subsystem
      mask Display:
      | plot(0.5+cos(linspace(0,2*pi,65))*0.3,0.5+sin(linspace(0,2*pi,65))*0.3);
      | plot([.29 .71],[.29 .71]);
      | plot([.71 .29],[.29 .71]);
  transposeQuaternion : Subsystem  mask(transposeQuaternion){}
      mask help:
      | Compute the transpose (inverse or conjugate) of the input quaternion
      |
      | Inputs:
      |   q     Quaternion
      |
      | Outputs:
      |   qt     Transpose of the input quaternion
      mask Help: eval('starDoc simulink/transposeQuaternion');
      mask Display: disp('q''');
  vB : Outport
  wires:
  Product/1 -> vB/1
  quat product1/1(q1*q2) -> Demux/1
  quat product/1(q1*q2) -> quat product1/1(q1)
  Mux/1 -> quat product/2(q2)
  transposeQuaternion/1(q') -> quat product/1(q1)
  qA2B/1 -> quat product1/2(q2), transposeQuaternion/1(q)
  vA/1 -> Mux/2
  Constant/1 -> Mux/1
  Demux/1 -> Product/1
  Demux/2 -> Product/2

== system attitude3d/frame2quat1 ==
  xB/A : Inport  PortDimensions=3
  yB/A : Inport  Port=2  PortDimensions=3
  zB/A : Inport  Port=3  PortDimensions=3
  MATLAB Function : MATLAB Function  TreatAsAtomicUnit=on
  qA2B : Outport  PortDimensions=4
  wires:
  xB/A/1 -> MATLAB Function/1(xB)
  yB/A/1 -> MATLAB Function/2(yB)
  zB/A/1 -> MATLAB Function/3(zB)
  MATLAB Function/1(qA2B) -> qA2B/1

== system attitude3d/quat2eul (small angles)1 ==
  dq : Inport  PortDimensions=4
  Demux : Demux  Outputs=[1 3]
  Gain : Gain  Gain=2
  manage quat sign : Switch  Criteria=u2 > Threshold
  take opposite : Gain  Gain=-1
  de : Outport  PortDimensions=3
  wires:
  manage quat sign/1 -> Gain/1
  take opposite/1 -> manage quat sign/3
  Demux/2 -> take opposite/1, manage quat sign/1
  Demux/1 -> manage quat sign/2  "scalar"
  dq/1 -> Demux/1
  Gain/1 -> de/1

== system attitude3d/quat2rot ==
  q_AB : Inport  PortDimensions=4
  Constant : Constant
  Demux : Demux  Outputs=[1 3]
  Divide : Product  Inputs=***
  Divide1 : Product  Inputs=/
  Divide2 : Product  Inputs=**
  Gain : Gain  Gain=2
  Norm : Subsystem  mask(Norm){}
      mask help: Computes the norm of a vector : y = ||u||.
      mask Help: eval('AstrolibHelp');
      mask Display: disp('||X||');
  Sign : Signum  ZeroCross=off
  Switch : Switch  Criteria=u2 ~= 0  ZeroCross=off
  Trigonometric Function : Trigonometry  Operator=atan2
  angleB2A : Outport  PortDimensions=1
  vector_A : Outport  Port=2  PortDimensions=3
  wires:
  Sign/1 -> Divide2/2, Divide/1
  Divide2/1 -> Trigonometric Function/2
  Divide1/1 -> Divide/3
  q_AB/1 -> Demux/1
  Demux/1 -> Divide2/1, Sign/1
  Demux/2 -> Norm/1(X), Divide/2
  Trigonometric Function/1 -> Gain/1
  Gain/1 -> angleB2A/1
  Divide/1 -> vector_A/1
  Norm/1(||X||) -> Trigonometric Function/1, Switch/1, Switch/2
  Switch/1 -> Divide1/1
  Constant/1 -> Switch/3

== system attitude3d/transposeQuaternion1 ==
  q : Inport  PortDimensions=4
  Gain1 : Gain  Gain=[1 -1 -1 -1]  SaturateOnIntegerOverflow=on  OutDataTypeStr=Inherit: Same as input  ParamDataTypeStr=Inherit: Same as input
  q' : Outport  PortDimensions=4
  wires:
  q/1 -> Gain1/1
  Gain1/1 -> q'/1

== system attitude3d/frame change/quat product ==
  q1 : Inport
  q2 : Inport  Port=2
  Cross Product : Subsystem  Tag=68  mask(CrossProduct){}
      mask help: Compute the cross product of two 3-vectors : y = u1 x u2
      mask Display:
      | plot([.4 .6],[.4 .6]);
      | plot([.6 .4],[.4 .6]);
  Demux : Demux  Outputs=[1 3]
  Demux1 : Demux  Outputs=[1 3]
  Dot Product : DotProduct  InputSameDT=on  OutDataTypeStr=Inherit: Inherit via internal rule
  Mux : Mux  Inputs=2
  Product : Product  SaturateOnIntegerOverflow=on  OutDataTypeStr=Inherit: Same as first input
  Product1 : Product  SaturateOnIntegerOverflow=on  OutDataTypeStr=Inherit: Same as first input
  Product2 : Product  SaturateOnIntegerOverflow=on  OutDataTypeStr=Inherit: Same as first input
  Sum : Sum  Inputs=+++  SaturateOnIntegerOverflow=on
  Sum1 : Sum  Inputs=|+-  SaturateOnIntegerOverflow=on
  q1*q2 : Outport
  wires:
  Demux/2 -> Product1/2, Cross Product/1(u1), Dot Product/2
  Demux/1 -> Product/1, Product2/1
  Demux1/1 -> Product1/1, Product2/2
  Demux1/2 -> Cross Product/2(u2), Product/2, Dot Product/1
  Cross Product/1(u1xu2) -> Sum/2
  Product/1 -> Sum/1
  Product1/1 -> Sum/3
  Sum/1 -> Mux/2  "vector"
  Product2/1 -> Sum1/1
  Dot Product/1 -> Sum1/2
  Sum1/1 -> Mux/1  "scalar"
  q1/1 -> Demux/1
  Mux/1 -> q1*q2/1
  q2/1 -> Demux1/1

== system attitude3d/frame change/quat product1 ==
  q1 : Inport
  q2 : Inport  Port=2
  Cross Product : Subsystem  Tag=68  mask(CrossProduct){}
      mask help: Compute the cross product of two 3-vectors : y = u1 x u2
      mask Display:
      | plot([.4 .6],[.4 .6]);
      | plot([.6 .4],[.4 .6]);
  Demux : Demux  Outputs=[1 3]
  Demux1 : Demux  Outputs=[1 3]
  Dot Product : DotProduct  InputSameDT=on  OutDataTypeStr=Inherit: Inherit via internal rule
  Mux : Mux  Inputs=2
  Product : Product  SaturateOnIntegerOverflow=on  OutDataTypeStr=Inherit: Same as first input
  Product1 : Product  SaturateOnIntegerOverflow=on  OutDataTypeStr=Inherit: Same as first input
  Product2 : Product  SaturateOnIntegerOverflow=on  OutDataTypeStr=Inherit: Same as first input
  Sum : Sum  Inputs=+++  SaturateOnIntegerOverflow=on
  Sum1 : Sum  Inputs=|+-  SaturateOnIntegerOverflow=on
  q1*q2 : Outport
  wires:
  q2/1 -> Demux1/1
  Mux/1 -> q1*q2/1
  q1/1 -> Demux/1
  Sum1/1 -> Mux/1  "scalar"
  Dot Product/1 -> Sum1/2
  Product2/1 -> Sum1/1
  Sum/1 -> Mux/2  "vector"
  Product1/1 -> Sum/3
  Product/1 -> Sum/1
  Cross Product/1(u1xu2) -> Sum/2
  Demux1/2 -> Dot Product/1, Product/2, Cross Product/2(u2)
  Demux1/1 -> Product2/2, Product1/1
  Demux/1 -> Product2/1, Product/1
  Demux/2 -> Dot Product/2, Cross Product/1(u1), Product1/2

== system attitude3d/frame change/transposeQuaternion ==
  q : Inport
  Gain1 : Gain  Gain=[1 -1 -1 -1]  SaturateOnIntegerOverflow=on  OutDataTypeStr=Inherit: Same as input  ParamDataTypeStr=Inherit: Same as input
  q' : Outport
  wires:
  q/1 -> Gain1/1
  Gain1/1 -> q'/1

== system attitude3d/frame change1/quat product ==
  q1 : Inport
  q2 : Inport  Port=2
  Cross Product : Subsystem  Tag=68  mask(CrossProduct){}
      mask help: Compute the cross product of two 3-vectors : y = u1 x u2
      mask Display:
      | plot([.4 .6],[.4 .6]);
      | plot([.6 .4],[.4 .6]);
  Demux : Demux  Outputs=[1 3]
  Demux1 : Demux  Outputs=[1 3]
  Dot Product : DotProduct  InputSameDT=on  OutDataTypeStr=Inherit: Inherit via internal rule
  Mux : Mux  Inputs=2
  Product : Product  SaturateOnIntegerOverflow=on  OutDataTypeStr=Inherit: Same as first input
  Product1 : Product  SaturateOnIntegerOverflow=on  OutDataTypeStr=Inherit: Same as first input
  Product2 : Product  SaturateOnIntegerOverflow=on  OutDataTypeStr=Inherit: Same as first input
  Sum : Sum  Inputs=+++  SaturateOnIntegerOverflow=on
  Sum1 : Sum  Inputs=|+-  SaturateOnIntegerOverflow=on
  q1*q2 : Outport
  wires:
  Demux/2 -> Product1/2, Cross Product/1(u1), Dot Product/2
  Demux/1 -> Product/1, Product2/1
  Demux1/1 -> Product1/1, Product2/2
  Demux1/2 -> Cross Product/2(u2), Product/2, Dot Product/1
  Cross Product/1(u1xu2) -> Sum/2
  Product/1 -> Sum/1
  Product1/1 -> Sum/3
  Sum/1 -> Mux/2  "vector"
  Product2/1 -> Sum1/1
  Dot Product/1 -> Sum1/2
  Sum1/1 -> Mux/1  "scalar"
  q1/1 -> Demux/1
  Mux/1 -> q1*q2/1
  q2/1 -> Demux1/1

== system attitude3d/frame change1/quat product1 ==
  q1 : Inport
  q2 : Inport  Port=2
  Cross Product : Subsystem  Tag=68  mask(CrossProduct){}
      mask help: Compute the cross product of two 3-vectors : y = u1 x u2
      mask Display:
      | plot([.4 .6],[.4 .6]);
      | plot([.6 .4],[.4 .6]);
  Demux : Demux  Outputs=[1 3]
  Demux1 : Demux  Outputs=[1 3]
  Dot Product : DotProduct  InputSameDT=on  OutDataTypeStr=Inherit: Inherit via internal rule
  Mux : Mux  Inputs=2
  Product : Product  SaturateOnIntegerOverflow=on  OutDataTypeStr=Inherit: Same as first input
  Product1 : Product  SaturateOnIntegerOverflow=on  OutDataTypeStr=Inherit: Same as first input
  Product2 : Product  SaturateOnIntegerOverflow=on  OutDataTypeStr=Inherit: Same as first input
  Sum : Sum  Inputs=+++  SaturateOnIntegerOverflow=on
  Sum1 : Sum  Inputs=|+-  SaturateOnIntegerOverflow=on
  q1*q2 : Outport
  wires:
  q2/1 -> Demux1/1
  Mux/1 -> q1*q2/1
  q1/1 -> Demux/1
  Sum1/1 -> Mux/1  "scalar"
  Dot Product/1 -> Sum1/2
  Product2/1 -> Sum1/1
  Sum/1 -> Mux/2  "vector"
  Product1/1 -> Sum/3
  Product/1 -> Sum/1
  Cross Product/1(u1xu2) -> Sum/2
  Demux1/2 -> Dot Product/1, Product/2, Cross Product/2(u2)
  Demux1/1 -> Product2/2, Product1/1
  Demux/1 -> Product2/1, Product/1
  Demux/2 -> Dot Product/2, Cross Product/1(u1), Product1/2

== system attitude3d/frame change1/transposeQuaternion ==
  q : Inport
  Gain1 : Gain  Gain=[1 -1 -1 -1]  SaturateOnIntegerOverflow=on  OutDataTypeStr=Inherit: Same as input  ParamDataTypeStr=Inherit: Same as input
  q' : Outport
  wires:
  q/1 -> Gain1/1
  Gain1/1 -> q'/1

== system attitude3d/frame change2/quat product ==
  q1 : Inport
  q2 : Inport  Port=2
  Cross Product : Subsystem  Tag=68  mask(CrossProduct){}
      mask help: Compute the cross product of two 3-vectors : y = u1 x u2
      mask Display:
      | plot([.4 .6],[.4 .6]);
      | plot([.6 .4],[.4 .6]);
  Demux : Demux  Outputs=[1 3]
  Demux1 : Demux  Outputs=[1 3]
  Dot Product : DotProduct  InputSameDT=on  OutDataTypeStr=Inherit: Inherit via internal rule
  Mux : Mux  Inputs=2
  Product : Product  SaturateOnIntegerOverflow=on  OutDataTypeStr=Inherit: Same as first input
  Product1 : Product  SaturateOnIntegerOverflow=on  OutDataTypeStr=Inherit: Same as first input
  Product2 : Product  SaturateOnIntegerOverflow=on  OutDataTypeStr=Inherit: Same as first input
  Sum : Sum  Inputs=+++  SaturateOnIntegerOverflow=on
  Sum1 : Sum  Inputs=|+-  SaturateOnIntegerOverflow=on
  q1*q2 : Outport
  wires:
  Demux/2 -> Product1/2, Cross Product/1(u1), Dot Product/2
  Demux/1 -> Product/1, Product2/1
  Demux1/1 -> Product1/1, Product2/2
  Demux1/2 -> Cross Product/2(u2), Product/2, Dot Product/1
  Cross Product/1(u1xu2) -> Sum/2
  Product/1 -> Sum/1
  Product1/1 -> Sum/3
  Sum/1 -> Mux/2  "vector"
  Product2/1 -> Sum1/1
  Dot Product/1 -> Sum1/2
  Sum1/1 -> Mux/1  "scalar"
  q1/1 -> Demux/1
  Mux/1 -> q1*q2/1
  q2/1 -> Demux1/1

== system attitude3d/frame change2/quat product1 ==
  q1 : Inport
  q2 : Inport  Port=2
  Cross Product : Subsystem  Tag=68  mask(CrossProduct){}
      mask help: Compute the cross product of two 3-vectors : y = u1 x u2
      mask Display:
      | plot([.4 .6],[.4 .6]);
      | plot([.6 .4],[.4 .6]);
  Demux : Demux  Outputs=[1 3]
  Demux1 : Demux  Outputs=[1 3]
  Dot Product : DotProduct  InputSameDT=on  OutDataTypeStr=Inherit: Inherit via internal rule
  Mux : Mux  Inputs=2
  Product : Product  SaturateOnIntegerOverflow=on  OutDataTypeStr=Inherit: Same as first input
  Product1 : Product  SaturateOnIntegerOverflow=on  OutDataTypeStr=Inherit: Same as first input
  Product2 : Product  SaturateOnIntegerOverflow=on  OutDataTypeStr=Inherit: Same as first input
  Sum : Sum  Inputs=+++  SaturateOnIntegerOverflow=on
  Sum1 : Sum  Inputs=|+-  SaturateOnIntegerOverflow=on
  q1*q2 : Outport
  wires:
  q2/1 -> Demux1/1
  Mux/1 -> q1*q2/1
  q1/1 -> Demux/1
  Sum1/1 -> Mux/1  "scalar"
  Dot Product/1 -> Sum1/2
  Product2/1 -> Sum1/1
  Sum/1 -> Mux/2  "vector"
  Product1/1 -> Sum/3
  Product/1 -> Sum/1
  Cross Product/1(u1xu2) -> Sum/2
  Demux1/2 -> Dot Product/1, Product/2, Cross Product/2(u2)
  Demux1/1 -> Product2/2, Product1/1
  Demux/1 -> Product2/1, Product/1
  Demux/2 -> Dot Product/2, Cross Product/1(u1), Product1/2

== system attitude3d/frame change2/transposeQuaternion ==
  q : Inport
  Gain1 : Gain  Gain=[1 -1 -1 -1]  SaturateOnIntegerOverflow=on  OutDataTypeStr=Inherit: Same as input  ParamDataTypeStr=Inherit: Same as input
  q' : Outport
  wires:
  q/1 -> Gain1/1
  Gain1/1 -> q'/1

== system attitude3d/frame change3/quat product ==
  q1 : Inport
  q2 : Inport  Port=2
  Cross Product : Subsystem  Tag=68  mask(CrossProduct){}
      mask help: Compute the cross product of two 3-vectors : y = u1 x u2
      mask Display:
      | plot([.4 .6],[.4 .6]);
      | plot([.6 .4],[.4 .6]);
  Demux : Demux  Outputs=[1 3]
  Demux1 : Demux  Outputs=[1 3]
  Dot Product : DotProduct  InputSameDT=on  OutDataTypeStr=Inherit: Inherit via internal rule
  Mux : Mux  Inputs=2
  Product : Product  SaturateOnIntegerOverflow=on  OutDataTypeStr=Inherit: Same as first input
  Product1 : Product  SaturateOnIntegerOverflow=on  OutDataTypeStr=Inherit: Same as first input
  Product2 : Product  SaturateOnIntegerOverflow=on  OutDataTypeStr=Inherit: Same as first input
  Sum : Sum  Inputs=+++  SaturateOnIntegerOverflow=on
  Sum1 : Sum  Inputs=|+-  SaturateOnIntegerOverflow=on
  q1*q2 : Outport
  wires:
  Demux/2 -> Product1/2, Cross Product/1(u1), Dot Product/2
  Demux/1 -> Product/1, Product2/1
  Demux1/1 -> Product1/1, Product2/2
  Demux1/2 -> Cross Product/2(u2), Product/2, Dot Product/1
  Cross Product/1(u1xu2) -> Sum/2
  Product/1 -> Sum/1
  Product1/1 -> Sum/3
  Sum/1 -> Mux/2  "vector"
  Product2/1 -> Sum1/1
  Dot Product/1 -> Sum1/2
  Sum1/1 -> Mux/1  "scalar"
  q1/1 -> Demux/1
  Mux/1 -> q1*q2/1
  q2/1 -> Demux1/1

== system attitude3d/frame change3/quat product1 ==
  q1 : Inport
  q2 : Inport  Port=2
  Cross Product : Subsystem  Tag=68  mask(CrossProduct){}
      mask help: Compute the cross product of two 3-vectors : y = u1 x u2
      mask Display:
      | plot([.4 .6],[.4 .6]);
      | plot([.6 .4],[.4 .6]);
  Demux : Demux  Outputs=[1 3]
  Demux1 : Demux  Outputs=[1 3]
  Dot Product : DotProduct  InputSameDT=on  OutDataTypeStr=Inherit: Inherit via internal rule
  Mux : Mux  Inputs=2
  Product : Product  SaturateOnIntegerOverflow=on  OutDataTypeStr=Inherit: Same as first input
  Product1 : Product  SaturateOnIntegerOverflow=on  OutDataTypeStr=Inherit: Same as first input
  Product2 : Product  SaturateOnIntegerOverflow=on  OutDataTypeStr=Inherit: Same as first input
  Sum : Sum  Inputs=+++  SaturateOnIntegerOverflow=on
  Sum1 : Sum  Inputs=|+-  SaturateOnIntegerOverflow=on
  q1*q2 : Outport
  wires:
  q2/1 -> Demux1/1
  Mux/1 -> q1*q2/1
  q1/1 -> Demux/1
  Sum1/1 -> Mux/1  "scalar"
  Dot Product/1 -> Sum1/2
  Product2/1 -> Sum1/1
  Sum/1 -> Mux/2  "vector"
  Product1/1 -> Sum/3
  Product/1 -> Sum/1
  Cross Product/1(u1xu2) -> Sum/2
  Demux1/2 -> Dot Product/1, Product/2, Cross Product/2(u2)
  Demux1/1 -> Product2/2, Product1/1
  Demux/1 -> Product2/1, Product/1
  Demux/2 -> Dot Product/2, Cross Product/1(u1), Product1/2

== system attitude3d/frame change3/transposeQuaternion ==
  q : Inport
  Gain1 : Gain  Gain=[1 -1 -1 -1]  SaturateOnIntegerOverflow=on  OutDataTypeStr=Inherit: Same as input  ParamDataTypeStr=Inherit: Same as input
  q' : Outport
  wires:
  q/1 -> Gain1/1
  Gain1/1 -> q'/1

== system attitude3d/frame change4/quat product ==
  q1 : Inport
  q2 : Inport  Port=2
  Cross Product : Subsystem  Tag=68  mask(CrossProduct){}
      mask help: Compute the cross product of two 3-vectors : y = u1 x u2
      mask Display:
      | plot([.4 .6],[.4 .6]);
      | plot([.6 .4],[.4 .6]);
  Demux : Demux  Outputs=[1 3]
  Demux1 : Demux  Outputs=[1 3]
  Dot Product : DotProduct  InputSameDT=on  OutDataTypeStr=Inherit: Inherit via internal rule
  Mux : Mux  Inputs=2
  Product : Product  SaturateOnIntegerOverflow=on  OutDataTypeStr=Inherit: Same as first input
  Product1 : Product  SaturateOnIntegerOverflow=on  OutDataTypeStr=Inherit: Same as first input
  Product2 : Product  SaturateOnIntegerOverflow=on  OutDataTypeStr=Inherit: Same as first input
  Sum : Sum  Inputs=+++  SaturateOnIntegerOverflow=on
  Sum1 : Sum  Inputs=|+-  SaturateOnIntegerOverflow=on
  q1*q2 : Outport
  wires:
  Demux/2 -> Product1/2, Cross Product/1(u1), Dot Product/2
  Demux/1 -> Product/1, Product2/1
  Demux1/1 -> Product1/1, Product2/2
  Demux1/2 -> Cross Product/2(u2), Product/2, Dot Product/1
  Cross Product/1(u1xu2) -> Sum/2
  Product/1 -> Sum/1
  Product1/1 -> Sum/3
  Sum/1 -> Mux/2  "vector"
  Product2/1 -> Sum1/1
  Dot Product/1 -> Sum1/2
  Sum1/1 -> Mux/1  "scalar"
  q1/1 -> Demux/1
  Mux/1 -> q1*q2/1
  q2/1 -> Demux1/1

== system attitude3d/frame change4/quat product1 ==
  q1 : Inport
  q2 : Inport  Port=2
  Cross Product : Subsystem  Tag=68  mask(CrossProduct){}
      mask help: Compute the cross product of two 3-vectors : y = u1 x u2
      mask Display:
      | plot([.4 .6],[.4 .6]);
      | plot([.6 .4],[.4 .6]);
  Demux : Demux  Outputs=[1 3]
  Demux1 : Demux  Outputs=[1 3]
  Dot Product : DotProduct  InputSameDT=on  OutDataTypeStr=Inherit: Inherit via internal rule
  Mux : Mux  Inputs=2
  Product : Product  SaturateOnIntegerOverflow=on  OutDataTypeStr=Inherit: Same as first input
  Product1 : Product  SaturateOnIntegerOverflow=on  OutDataTypeStr=Inherit: Same as first input
  Product2 : Product  SaturateOnIntegerOverflow=on  OutDataTypeStr=Inherit: Same as first input
  Sum : Sum  Inputs=+++  SaturateOnIntegerOverflow=on
  Sum1 : Sum  Inputs=|+-  SaturateOnIntegerOverflow=on
  q1*q2 : Outport
  wires:
  q2/1 -> Demux1/1
  Mux/1 -> q1*q2/1
  q1/1 -> Demux/1
  Sum1/1 -> Mux/1  "scalar"
  Dot Product/1 -> Sum1/2
  Product2/1 -> Sum1/1
  Sum/1 -> Mux/2  "vector"
  Product1/1 -> Sum/3
  Product/1 -> Sum/1
  Cross Product/1(u1xu2) -> Sum/2
  Demux1/2 -> Dot Product/1, Product/2, Cross Product/2(u2)
  Demux1/1 -> Product2/2, Product1/1
  Demux/1 -> Product2/1, Product/1
  Demux/2 -> Dot Product/2, Cross Product/1(u1), Product1/2
